simulink model "ddc_simulink_CRD_fixed"  (R2022b)
settings: Solver=FixedStepAuto  StartTime=0.0  StopTime=0.005  RelTol=1e-3
values from neighbouring files (symbols this model uses):
  Fs = 60000000    [workspace.mat]
  h = [0 -0.000623274929429 -0.00453372620191 -0.00853119631049 0.00761421992952 0.0709963150011 0.17516404115 0.259913621361 0.259913621361 0.17516404115 0.0709963150011 0.00761421992952 ... (16 elements, 1x16)]    [workspace.mat]
  N = 31    [workspace.mat]
  T = 2e-05    [workspace.mat]
  Ts = 1.66666666667e-08    [workspace.mat]
libraries: dsphdlsigops2 x2, simulink x1
settings Model: MinMaxOverflowLogging=MinMaxAndOverflow  FPTRunName=BaselineRun  FPTShortcutValueString='{{},{''BaselineRun'',1,1,1,''BaselineRun'','''',{},''M'','''',''''},{''EmbeddedRun'',1,1,1,''EmbeddedRun'','''',{},''M'','''',''''}}'  Creator=caleb  LastModifiedBy=caleb
settings DebuggingCC: SignalRangeChecking=warning

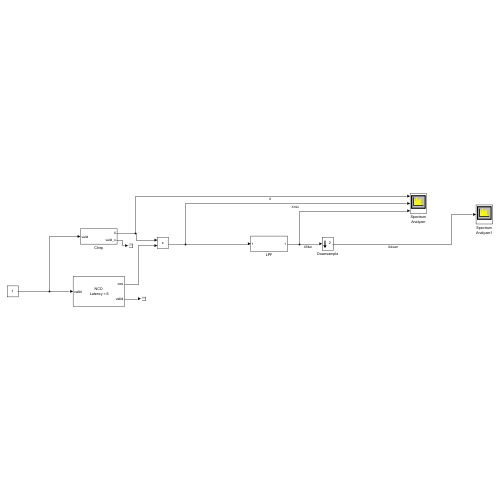
[thumbnail: Simulink's stored preview of the top-level diagram]
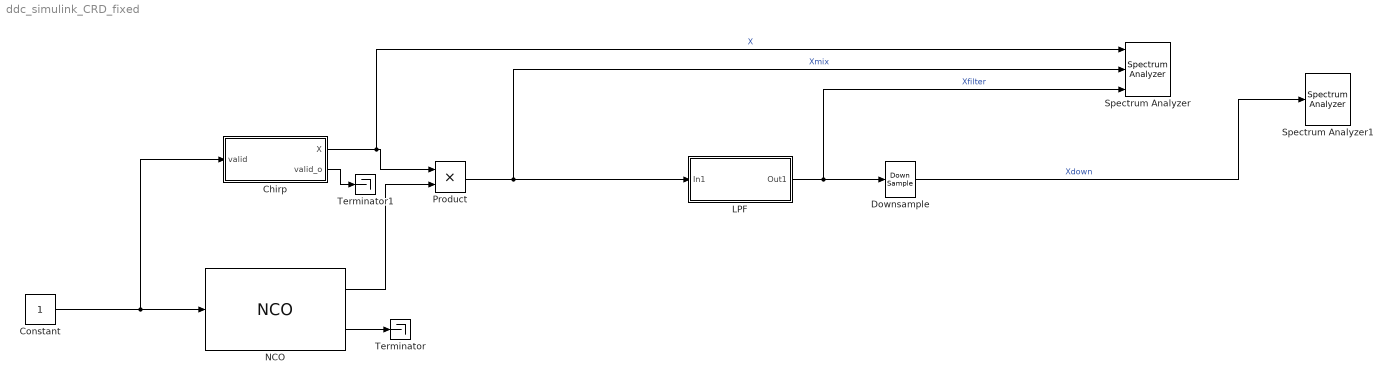
== system ddc_simulink_CRD_fixed ==
  Chirp : Subsystem
  Constant : Constant  OutDataTypeStr=boolean  SampleTime=Ts
  Downsample : DownSample  RateOptions=Allow multirate processing
  LPF : Subsystem
  NCO : dsphdlsigops2/NCO  PhaseIncrementSource=Property  PhaseIncrement=phIncr  PhaseOffsetSource=Property  PhaseOffset=phOff  DitherSource=Property  NumDitherBits=ditherBits  SamplesPerFrame=1  LUTCompress=off  ResetAction=off  Waveform=Cosine  PhasePort=off  SimulateUsing=Code generation  AccumulatorWL=N  PhaseQuantization=on  NumQuantizerAccumulatorBits=Q  OutputDataType=Binary point scaling  OutputWL=16  OutputFL=14
  Product : Product  OutDataTypeStr=fixdt(1,16,14)
  Spectrum Analyzer : SpectrumAnalyzer  NumInputPorts=3
  Spectrum Analyzer1 : SpectrumAnalyzer
  Terminator : Terminator
  Terminator1 : Terminator
  wires:
  Constant/1 -> Chirp/1(valid), NCO/1
  NCO/1 -> Product/2
  Product/1 -> Spectrum Analyzer/2, LPF/1(In1)  "Xmix"
  LPF/1(Out1) -> Downsample/1, Spectrum Analyzer/3  "Xfilter"
  Downsample/1 -> Spectrum Analyzer1/1  "Xdown"
  NCO/2 -> Terminator/1
  Chirp/1(X) -> Spectrum Analyzer/1, Product/1  "X"
  Chirp/2(valid_o) -> Terminator1/1

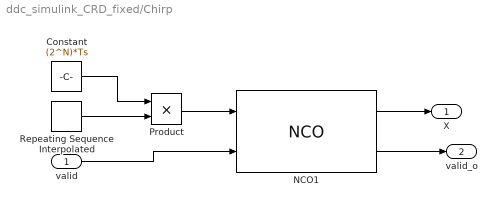
== system ddc_simulink_CRD_fixed/Chirp ==
  valid : Inport
  Constant : Constant  Value=(2^N)*Ts
  NCO1 : dsphdlsigops2/NCO  PhaseIncrementSource=Input port  PhaseIncrement=phIncr  PhaseOffsetSource=Property  PhaseOffset=phOff  DitherSource=Property  NumDitherBits=ditherBits  SamplesPerFrame=1  LUTCompress=off  ResetAction=off  Waveform=Cosine  PhasePort=off  SimulateUsing=Code generation  AccumulatorWL=N  PhaseQuantization=on  NumQuantizerAccumulatorBits=Q  OutputDataType=Binary point scaling  OutputWL=16  OutputFL=14
  Product : Product
  Repeating Sequence Interpolated : simulink/Sources/Repeating Sequence Interpolated  OutValues=[10e6 20e6].'  TimeValues=[0 T].'  LookUpMeth=Interpolation-Use End Values  tsamp=1/Fs  OutMin=[]  OutMax=[]  OutDataTypeStr=double  OutputDataTypeScalingMode=double  OutDataType=fixdt(0,8)  OutScaling=2^-10
  X : Outport
  valid_o : Outport  Port=2
  wires:
  Product/1 -> NCO1/1
  Constant/1 -> Product/1
  Repeating Sequence Interpolated/1 -> Product/2
  valid/1 -> NCO1/2
  NCO1/2 -> valid_o/1
  NCO1/1 -> X/1

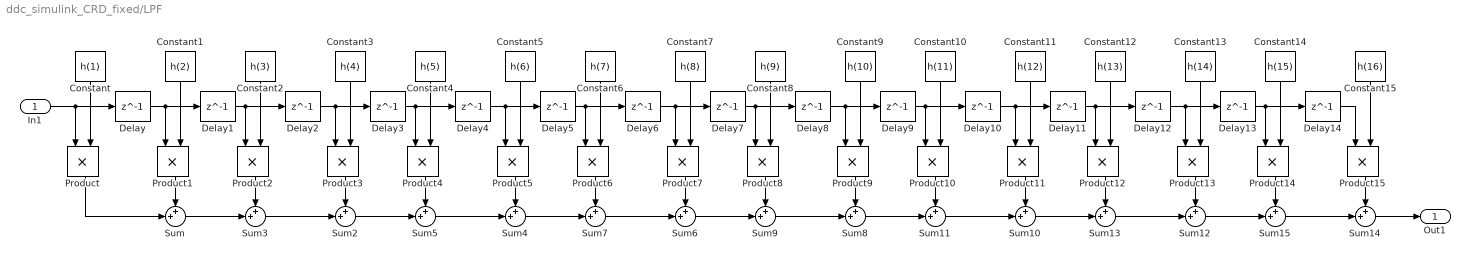
== system ddc_simulink_CRD_fixed/LPF ==
  In1 : Inport  OutDataTypeStr=fixdt(1,16,14)
  Constant : Constant  Value=h(1)  OutDataTypeStr=fixdt(1,16,4)
  Constant1 : Constant  Value=h(2)  OutDataTypeStr=fixdt(1,16,25)
  Constant10 : Constant  Value=h(11)  OutDataTypeStr=fixdt(0,16,19)
  Constant11 : Constant  Value=h(12)  OutDataTypeStr=fixdt(0,16,23)
  Constant12 : Constant  Value=h(13)  OutDataTypeStr=fixdt(1,16,21)
  Constant13 : Constant  Value=h(14)  OutDataTypeStr=fixdt(1,16,22)
  Constant14 : Constant  Value=h(15)  OutDataTypeStr=fixdt(1,16,25)
  Constant15 : Constant  Value=h(16)  OutDataTypeStr=fixdt(1,16,4)
  Constant2 : Constant  Value=h(3)  OutDataTypeStr=fixdt(1,16,22)
  Constant3 : Constant  Value=h(4)  OutDataTypeStr=fixdt(1,16,21)
  Constant4 : Constant  Value=h(5)  OutDataTypeStr=fixdt(0,16,23)
  Constant5 : Constant  Value=h(6)  OutDataTypeStr=fixdt(0,16,19)
  Constant6 : Constant  Value=h(7)  OutDataTypeStr=fixdt(0,16,18)
  Constant7 : Constant  Value=h(8)  OutDataTypeStr=fixdt(0,16,17)
  Constant8 : Constant  Value=h(9)  OutDataTypeStr=fixdt(0,16,17)
  Constant9 : Constant  Value=h(10)  OutDataTypeStr=fixdt(0,16,18)
  Delay{,1..14} (15 alike) : Delay  DelayLength=1  InitialCondition=0  UseCircularBuffer=on
  Product : Product  OutDataTypeStr=fixdt(1,16,4)
  Product1 : Product  OutDataTypeStr=fixdt(1,16,25)
  Product10 : Product  OutDataTypeStr=fixdt(1,16,18)
  Product{2,4,11,13} (4 alike) : Product  OutDataTypeStr=fixdt(1,16,22)
  Product12 : Product  OutDataTypeStr=fixdt(1,16,21)
  Product14 : Product  OutDataTypeStr=fixdt(1,16,25)
  Product15 : Product  OutDataTypeStr=fixdt(1,16,4)
  Product3 : Product  OutDataTypeStr=fixdt(1,16,21)
  Product5 : Product  OutDataTypeStr=fixdt(1,16,18)
  Product6 : Product  OutDataTypeStr=fixdt(1,16,17)
  Product7 : Product  OutDataTypeStr=fixdt(1,16,16)
  Product8 : Product  OutDataTypeStr=fixdt(1,16,16)
  Product9 : Product  OutDataTypeStr=fixdt(1,16,17)
  Sum : Sum  Inputs=++|  OutDataTypeStr=fixdt(1,16,25)
  Sum{6,8..15} (9 alike) : Sum  Inputs=++|  OutDataTypeStr=fixdt(1,16,16)
  Sum2 : Sum  Inputs=++|  OutDataTypeStr=fixdt(1,16,21)
  Sum3 : Sum  Inputs=++|  OutDataTypeStr=fixdt(1,16,22)
  Sum4 : Sum  Inputs=++|  OutDataTypeStr=fixdt(1,16,18)
  Sum5 : Sum  Inputs=++|  OutDataTypeStr=fixdt(1,16,21)
  Sum7 : Sum  Inputs=++|  OutDataTypeStr=fixdt(1,16,17)
  Out1 : Outport
  wires:
  In1/1 -> Delay/1, Product/1
  Delay/1 -> Product1/1, Delay1/1
  Constant/1 -> Product/2
  Constant1/1 -> Product1/2
  Product1/1 -> Sum/1
  Product/1 -> Sum/2
  Constant2/1 -> Product2/2
  Delay1/1 -> Delay2/1, Product2/1
  Product2/1 -> Sum3/1
  Delay2/1 -> Product3/1, Delay3/1
  Sum3/1 -> Sum2/2
  Constant3/1 -> Product3/2
  Product3/1 -> Sum2/1
  Constant4/1 -> Product4/2
  Delay3/1 -> Delay4/1, Product4/1
  Product4/1 -> Sum5/1
  Delay4/1 -> Product5/1, Delay5/1
  Sum5/1 -> Sum4/2
  Constant5/1 -> Product5/2
  Product5/1 -> Sum4/1
  Constant6/1 -> Product6/2
  Delay5/1 -> Delay6/1, Product6/1
  Product6/1 -> Sum7/1
  Delay6/1 -> Product7/1, Delay7/1
  Sum7/1 -> Sum6/2
  Constant7/1 -> Product7/2
  Product7/1 -> Sum6/1
  Constant8/1 -> Product8/2
  Delay7/1 -> Delay8/1, Product8/1
  Product8/1 -> Sum9/1
  Delay8/1 -> Product9/1, Delay9/1
  Sum9/1 -> Sum8/2
  Constant9/1 -> Product9/2
  Product9/1 -> Sum8/1
  Constant10/1 -> Product10/2
  Delay9/1 -> Delay10/1, Product10/1
  Product10/1 -> Sum11/1
  Delay10/1 -> Product11/1, Delay11/1
  Sum11/1 -> Sum10/2
  Constant11/1 -> Product11/2
  Product11/1 -> Sum10/1
  Constant12/1 -> Product12/2
  Delay11/1 -> Delay12/1, Product12/1
  Product12/1 -> Sum13/1
  Delay12/1 -> Product13/1, Delay13/1
  Sum13/1 -> Sum12/2
  Constant13/1 -> Product13/2
  Product13/1 -> Sum12/1
  Constant14/1 -> Product14/2
  Delay13/1 -> Delay14/1, Product14/1
  Product14/1 -> Sum15/1
  Delay14/1 -> Product15/1
  Sum15/1 -> Sum14/2
  Constant15/1 -> Product15/2
  Product15/1 -> Sum14/1
  Sum12/1 -> Sum15/2
  Sum10/1 -> Sum13/2
  Sum8/1 -> Sum11/2
  Sum6/1 -> Sum9/2
  Sum4/1 -> Sum7/2
  Sum2/1 -> Sum5/2
  Sum/1 -> Sum3/2
  Sum14/1 -> Out1/1
